simulink model "Non_ideal_swarming"  (R2023b)
settings: Solver=VariableStepAuto  StartTime=0.0  StopTime=10.0  RelTol=1e-3
libraries: dspstat3 x3, uavutilslib x2, sensorinslib x1
settings Model: Creator=rakshan  LastModifiedBy=rakshan
settings DebuggingCC: ParameterPrecisionLossMsg=none

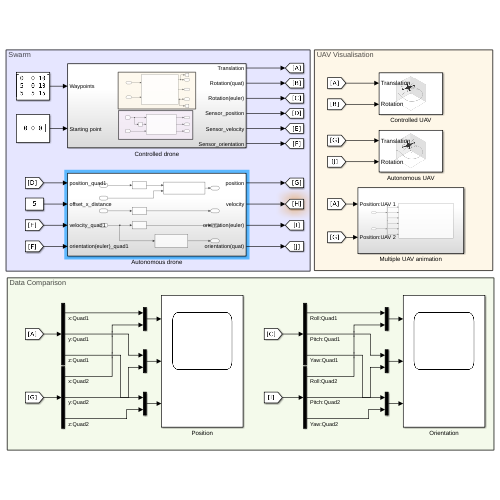
[thumbnail: Simulink's stored preview of the top-level diagram]
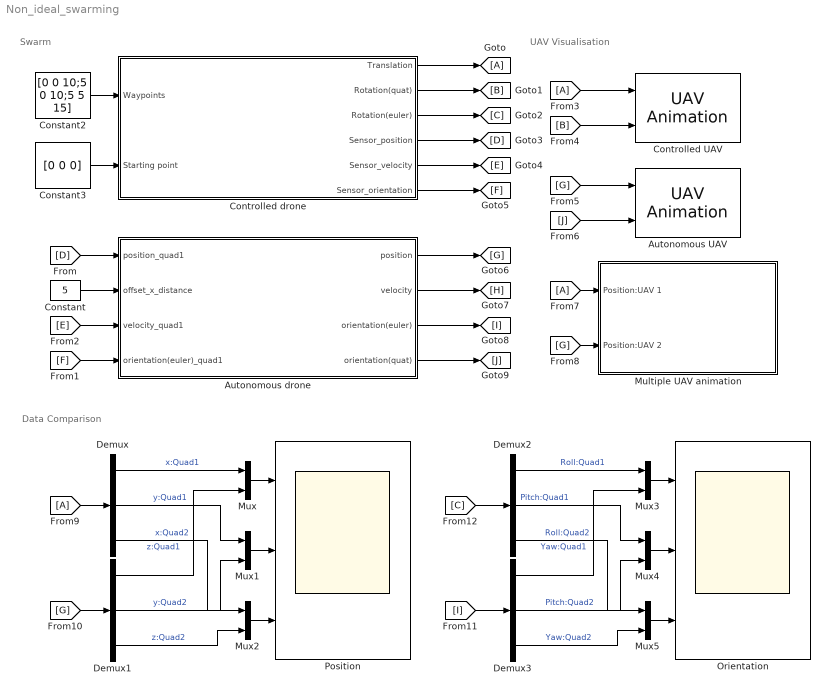
== system Non_ideal_swarming ==
  note: Data Comparison
  note: UAV Visualisation
  note: Swarm
  Autonomous UAV : uavutilslib/UAV Animation  UAVType=Multirotor  UAVSize=1  InertialZDirection=Up  SampleTime=-1
  Autonomous drone : Subsystem
  Constant : Constant  Value=5
  Constant2 : Constant  Value=[0 0 10;5 0 10;5 5 15]  VectorParams1D=off
  Constant3 : Constant  Value=[0 0 0]  VectorParams1D=off
  Controlled UAV : uavutilslib/UAV Animation  UAVType=Multirotor  UAVSize=1  InertialZDirection=Up  SampleTime=-1
  Controlled drone : Subsystem
  Demux{,1..3} (4 alike) : Demux  Outputs=3
  From3 : From
  From7 : From
  From9 : From
  Goto : Goto
  Multiple UAV animation : Subsystem
  Mux{,1..5} (6 alike) : Mux  Inputs=2
  Orientation : Scope  NumInputPorts=3
  Position : Scope  NumInputPorts=3
  wires:
  Controlled drone/1(Translation) -> Goto/1
  Controlled drone/2(Rotation(quat)) -> [B]
  Controlled drone/3(Rotation(euler)) -> [C]
  Controlled drone/4(Sensor_position) -> [D]
  Controlled drone/5(Sensor_velocity) -> [E]
  Controlled drone/6(Sensor_orientation) -> [F]
  Constant3/1 -> Controlled drone/2(Starting point)
  Constant2/1 -> Controlled drone/1(Waypoints)
  [D] -> Autonomous drone/1(position_quad1)
  Constant/1 -> Autonomous drone/2(offset_x_distance)
  [E] -> Autonomous drone/3(velocity_quad1)
  [F] -> Autonomous drone/4(orientation(euler)_quad1)
  Autonomous drone/1(position) -> [G]
  Autonomous drone/2(velocity) -> [H]
  Autonomous drone/3(orientation(euler)) -> [I]
  Autonomous drone/4(orientation(quat)) -> [J]
  From3/1 -> Controlled UAV/1
  [B] -> Controlled UAV/2
  [G] -> Autonomous UAV/1
  [J] -> Autonomous UAV/2
  From7/1 -> Multiple UAV animation/1(Position:UAV 1)
  [G] -> Multiple UAV animation/2(Position:UAV 2)
  From9/1 -> Demux/1
  Demux1/1 -> Mux/2  "x:Quad2"
  Demux1/2 -> Mux1/2  "y:Quad2"
  Demux1/3 -> Mux2/2  "z:Quad2"
  [G] -> Demux1/1
  Mux/1 -> Position/1
  Mux1/1 -> Position/2
  Mux2/1 -> Position/3
  Demux/1 -> Mux/1  "x:Quad1"
  Demux/2 -> Mux1/1  "y:Quad1"
  Demux/3 -> Mux2/1  "z:Quad1"
  Demux3/1 -> Mux3/2  "Roll:Quad2"
  Demux3/3 -> Mux5/2  "Yaw:Quad2"
  Demux2/1 -> Mux3/1  "Roll:Quad1"
  Mux5/1 -> Orientation/3
  [I] -> Demux3/1
  Mux3/1 -> Orientation/1
  Demux2/3 -> Mux5/1  "Yaw:Quad1"
  Demux2/2 -> Mux4/1  "Pitch:Quad1"
  Demux3/2 -> Mux4/2  "Pitch:Quad2"
  Mux4/1 -> Orientation/2
  [C] -> Demux2/1

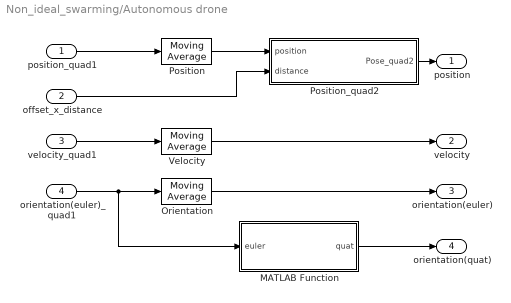
== system Non_ideal_swarming/Autonomous drone ==
  position_quad1 : Inport
  offset_x_distance : Inport  Port=2
  velocity_quad1 : Inport  Port=3
  orientation(euler)_quad1 : Inport  Port=4
  MATLAB Function : MATLAB Function  TreatAsAtomicUnit=on
  Orientation : dspstat3/Moving Average  Method=Exponential weighting  ForgettingFactorPort=off  SpecifyWindowLength=on  WindowLength=4  OverlapLength=3  AllowArbitraryInputLength=off  ForgettingFactor=0.9  SimulateUsing=Code generation
  Position : dspstat3/Moving Average  Method=Exponential weighting  ForgettingFactorPort=off  SpecifyWindowLength=on  WindowLength=4  OverlapLength=3  AllowArbitraryInputLength=off  ForgettingFactor=0.9  SimulateUsing=Code generation
  Position_quad2 : MATLAB Function  TreatAsAtomicUnit=on
  Velocity : dspstat3/Moving Average  Method=Exponential weighting  ForgettingFactorPort=off  SpecifyWindowLength=on  WindowLength=4  OverlapLength=3  AllowArbitraryInputLength=off  ForgettingFactor=0.9  SimulateUsing=Code generation
  position : Outport
  velocity : Outport  Port=2
  orientation(euler) : Outport  Port=3
  orientation(quat) : Outport  Port=4
  wires:
  Position/1 -> Position_quad2/1(position)
  offset_x_distance/1 -> Position_quad2/2(distance)
  Orientation/1 -> orientation(euler)/1
  velocity_quad1/1 -> Velocity/1
  Position_quad2/1(Pose_quad2) -> position/1
  orientation(euler)_quad1/1 -> MATLAB Function/1(euler), Orientation/1
  MATLAB Function/1(quat) -> orientation(quat)/1
  position_quad1/1 -> Position/1
  Velocity/1 -> velocity/1

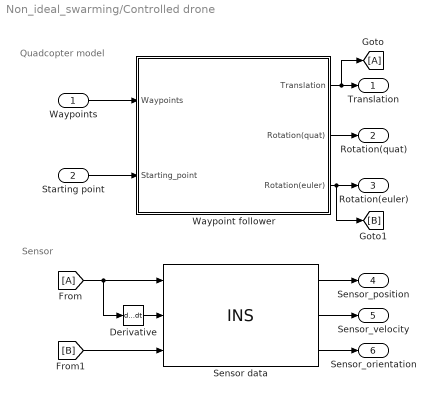
== system Non_ideal_swarming/Controlled drone ==
  note: Quadcopter model
  note: Sensor
  Waypoints : Inport
  Starting point : Inport  Port=2
  Derivative : Derivative
  From : From
  Goto : Goto
  Sensor data : sensorinslib/INS  MountingLocation=[0 0 0]  RollAccuracy=0.2  PitchAccuracy=0.2  YawAccuracy=1  PositionAccuracy=1  VelocityAccuracy=0.05  UseAccelAndAngVel=off  AccelerationAccuracy=0  AngularVelocityAccuracy=0  TimeInput=off  PositionErrorFactor=[0 0 0]  SeedDouble=67  SimulateUsing=Code generation
      settings: LibrarySourceBlock=drivingscenarioandsensors/INS
  Waypoint follower : Subsystem
  Translation : Outport
  Rotation(quat) : Outport  Port=2
  Rotation(euler) : Outport  Port=3
  Sensor_position : Outport  Port=4
  Sensor_velocity : Outport  Port=5
  Sensor_orientation : Outport  Port=6
  wires:
  Waypoint follower/3(Rotation(euler)) -> Rotation(euler)/1, [B]
  Sensor data/1 -> Sensor_position/1
  From/1 -> Derivative/1, Sensor data/1
  Starting point/1 -> Waypoint follower/2(Starting_point)
  Waypoints/1 -> Waypoint follower/1(Waypoints)
  Sensor data/2 -> Sensor_velocity/1
  Waypoint follower/2(Rotation(quat)) -> Rotation(quat)/1
  Derivative/1 -> Sensor data/2
  Sensor data/3 -> Sensor_orientation/1
  Waypoint follower/1(Translation) -> Goto/1, Translation/1
  [B] -> Sensor data/3

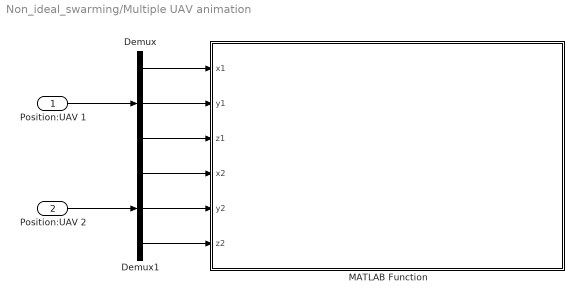
== system Non_ideal_swarming/Multiple UAV animation ==
  Position:UAV 1 : Inport
  Position:UAV 2 : Inport  Port=2
  Demux : Demux  Outputs=3
  Demux1 : Demux  Outputs=3
  MATLAB Function : MATLAB Function  TreatAsAtomicUnit=on
  wires:
  Demux/1 -> MATLAB Function/1(x1)
  Demux/2 -> MATLAB Function/2(y1)
  Demux/3 -> MATLAB Function/3(z1)
  Demux1/1 -> MATLAB Function/4(x2)
  Demux1/2 -> MATLAB Function/5(y2)
  Demux1/3 -> MATLAB Function/6(z2)
  Position:UAV 2/1 -> Demux1/1
  Position:UAV 1/1 -> Demux/1

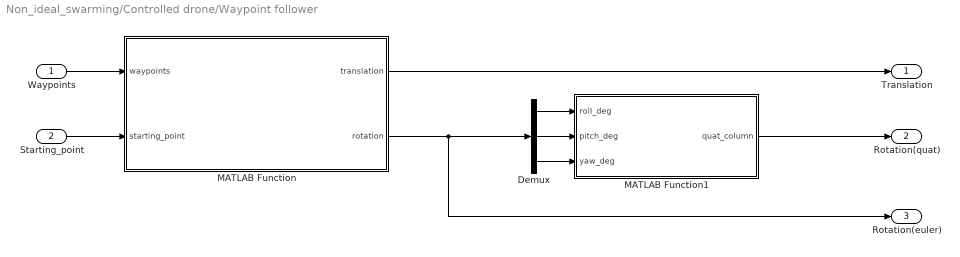
== system Non_ideal_swarming/Controlled drone/Waypoint follower ==
  Waypoints : Inport
  Starting_point : Inport  Port=2
  Demux : Demux  Outputs=3
  MATLAB Function : MATLAB Function  TreatAsAtomicUnit=on
  MATLAB Function1 : MATLAB Function  TreatAsAtomicUnit=on
  Translation : Outport
  Rotation(quat) : Outport  Port=2
  Rotation(euler) : Outport  Port=3
  wires:
  Demux/1 -> MATLAB Function1/1(roll_deg)
  Demux/3 -> MATLAB Function1/3(yaw_deg)
  Demux/2 -> MATLAB Function1/2(pitch_deg)
  MATLAB Function1/1(quat_column) -> Rotation(quat)/1
  MATLAB Function/2(rotation) -> Rotation(euler)/1, Demux/1
  Waypoints/1 -> MATLAB Function/1(waypoints)
  Starting_point/1 -> MATLAB Function/2(starting_point)
  MATLAB Function/1(translation) -> Translation/1

== matlab function Non_ideal_swarming/Controlled drone/Waypoint follower/MATLAB Function ==
  data: waypoints input; translation output; rotation output; starting_point input
function [translation, rotation] = interpolateWaypointsSimulink(waypoints,starting_point)
    persistent current_waypoint;
    persistent current_index;
    time_step = 0.4;
   
    waypoints = [starting_point;waypoints]
    % Initialize persistent variables on first call
    if isempty(current_waypoint)
        current_waypoint = waypoints(1,:);
        current_index = 1;
    end
    
    % Initialize outputs
    translation = zeros(1, 3);
    rotation = zeros(1, 3); % Euler angles: [yaw, pitch, roll]
    
    % Check if reached last waypoint
    if current_index == size(waypoints, 1)
        translation = waypoints(end, :);
        rotation = [0 0 0]; % No rotation (identity)
    else
        % Interpolate translation
        translation = current_waypoint;
        next_waypoint = waypoints(current_index + 1, :);
        current_waypoint = current_waypoint + (next_waypoint - current_waypoint) * time_step;
        
        % Calculate direction vector
        direction_vector = next_waypoint - current_waypoint;
        direction_vector = direction_vector / norm(direction_vector); % Normalize
        
        % Calculate rotation angles (Euler angles)
        yaw = atan2(direction_vector(2), direction_vector(1));
        pitch = asin(direction_vector(3));
        roll = 0; % Assuming no roll motion
        
        % Update rotation
        rotation = [yaw pitch roll];
        
        % Check if reached next waypoint
        if norm(current_waypoint - next_waypoint) < 0.01
            current_index = current_index + 1;
        end
    end
end

== matlab function Non_ideal_swarming/Autonomous drone/Position_quad2 ==
  data: position input; Pose_quad2 output; distance input
function Pose_quad2 = positionQuad(position, distance)
    % Extract the x, y, and z coordinates
    x = position(1);
    y = position(2);
    z = position(3);
    
    % Add 5 to the x-coordinate
    x = x + distance;
    
    % Create the new position vector
    Pose_quad2 = [x, y, z];
end

== matlab function Non_ideal_swarming/Controlled drone/Waypoint follower/MATLAB Function1 ==
  data: roll_deg input; quat_column output; pitch_deg input; yaw_deg input
function quat_column = eulerToQuat(roll_deg, pitch_deg, yaw_deg)
    % Convert Euler angles to radians
    roll_rad = deg2rad(roll_deg);
    pitch_rad = deg2rad(pitch_deg);
    yaw_rad = deg2rad(yaw_deg);

    % Calculate half angles
    roll_half = roll_rad / 2;
    pitch_half = pitch_rad / 2;
    yaw_half = yaw_rad / 2;

    % Calculate trigonometric functions
    roll_sin = sin(roll_half);
    roll_cos = cos(roll_half);
    pitch_sin = sin(pitch_half);
    pitch_cos = cos(pitch_half);
    yaw_sin = sin(yaw_half);
    yaw_cos = cos(yaw_half);

    % Calculate quaternion components
    q0 = roll_cos * pitch_cos * yaw_cos + roll_sin * pitch_sin * yaw_sin;
    q1 = roll_sin * pitch_cos * yaw_cos - roll_cos * pitch_sin * yaw_sin;
    q2 = roll_cos * pitch_sin * yaw_cos + roll_sin * pitch_cos * yaw_sin;
    q3 = roll_cos * pitch_cos * yaw_sin - roll_sin * pitch_sin * yaw_cos;

    % Format the quaternion as a column vector
    quat_column = [q0; q1; q2; q3];
end

== matlab function Non_ideal_swarming/Multiple UAV animation/MATLAB Function ==
  data: x1 input; y1 input; z1 input; x2 input; y2 input; z2 input
% uav_animation.m
function uav_animation(x1, y1, z1, x2, y2, z2)
    persistent traj_x1 traj_y1 traj_z1 traj_x2 traj_y2 traj_z2;
    
    % Initialize the figure
    figure(1);
    clf;
    hold on;
    axis equal;
    grid on;
    xlabel('X');
    ylabel('Y');
    zlabel('Z');
    legend;
    
    % Define a simple UAV shape (e.g., a cuboid)
    [x, y, z] = create_uav_shape();
    
    % Append current positions to the trajectory arrays
    if isempty(traj_x1)
        traj_x1 = x1;
        traj_y1 = y1;
        traj_z1 = z1;
        traj_x2 = x2;
        traj_y2 = y2;
        traj_z2 = z2;
    else
        traj_x1 = [traj_x1 x1];
        traj_y1 = [traj_y1 y1];
        traj_z1 = [traj_z1 z1];
        traj_x2 = [traj_x2 x2];
        traj_y2 = [traj_y2 y2];
        traj_z2 = [traj_z2 z2];
    end

    % Plot UAV1
    surf(x + x1, y + y1, z + z1, 'FaceColor', 'r', 'EdgeColor', 'none','DisplayName',"UAV 1");
    
    % Plot UAV2
    surf(x + x2, y + y2, z + z2, 'FaceColor', 'b', 'EdgeColor', 'none',"DisplayName","UAV 2");

    % Plot trajectory for UAV1
    plot3(traj_x1, traj_y1, traj_z1, '--r', 'LineWidth', 1, 'DisplayName', 'Trajectory: UAV 1');
    
    % Plot trajectory for UAV2
    plot3(traj_x2, traj_y2, traj_z2, '--b', 'LineWidth', 1, 'DisplayName', 'Trajectory: UAV 2');
    
    view(3); % Set the view to 3D
    drawnow;
end

function [x, y, z] = create_uav_shape()
    % Create a simple cuboid shape for the UAV
    [x, y, z] = ndgrid([-0.5, 0.5], [-0.5, 0.5], [-0.1, 0.1]);
    
    % Convert to surface coordinates
    x = reshape(x, [2, 2, 2]);
    y = reshape(y, [2, 2, 2]);
    z = reshape(z, [2, 2, 2]);

    % Create the faces of the cuboid
    x = [x(:, :, 1); x(:, :, 2)];
    y = [y(:, :, 1); y(:, :, 2)];
    z = [z(:, :, 1); z(:, :, 2)];
end

== matlab function Non_ideal_swarming/Autonomous drone/MATLAB Function ==
  data: euler input; quat output
function quat = eulerToQuaternion(euler)
    % Extract the roll, pitch, and yaw angles
    roll = euler(1);
    pitch = euler(2);
    yaw = euler(3);
    
    % Convert degrees to radians
    roll = deg2rad(roll);
    pitch = deg2rad(pitch);
    yaw = deg2rad(yaw);
    
    % Compute the quaternion components
    cy = cos(yaw * 0.5);
    sy = sin(yaw * 0.5);
    cp = cos(pitch * 0.5);
    sp = sin(pitch * 0.5);
    cr = cos(roll * 0.5);
    sr = sin(roll * 0.5);

    qw = cr * cp * cy + sr * sp * sy;
    qx = sr * cp * cy - cr * sp * sy;
    qy = cr * sp * cy + sr * cp * sy;
    qz = cr * cp * sy - sr * sp * cy;
    
    % Return the quaternion as a 4-element vector
    quat = [qw, qx, qy, qz];
end
